simulink model "Running_mex_SIMULINK_PID"  (R2020a)
settings: Solver=VariableStepAuto  StartTime=0.0  StopTime=inf  RelTol=1e-3
values from neighbouring files (symbols this model uses):
  angdes = [0 0 0]    [simulink_run_file.m]
  Kd = .105    (= 0.105)    [simulink_run_file.m]
  Kint = 0.01    [simulink_run_file.m]
  Kint_time = .5    (= 0.5)    [simulink_run_file.m]
  Kp = .065    (= 0.065)    [simulink_run_file.m]
  refresh = .005    (= 0.005)    [simulink_run_file.m]
  Tfinal_master = refresh*NumSteps    [simulink_run_file.m]
  Tmax = 2/1000    (= 0.002)    [simulink_run_file.m]
undefined symbols (not defined in the file or in its folder): get_initial_inputs
settings Model: Creator=hoddid  LastModifiedBy=hoddid

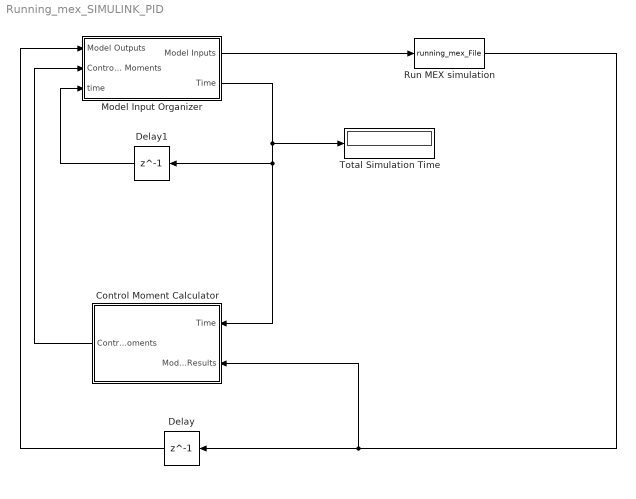
== system Running_mex_SIMULINK_PID ==
  Control Moment Calculator : Subsystem
  Delay : Delay  DelayLength=1
  Delay1 : Delay  DelayLength=1
  Model Input Organizer : Subsystem
  Run MEX simulation : MATLABFcn  MATLABFcn=running_mex_File  OutputDimensions=[1 32]  Output1D=off
  Total Simulation Time : Display
  wires:
  Model Input Organizer/1(Model Inputs) -> Run MEX simulation/1
  Delay/1 -> Model Input Organizer/1(Model Outputs)
  Delay1/1 -> Model Input Organizer/3(time)
  Control Moment Calculator/1(Control Moments) -> Model Input Organizer/2(Control Moments)
  Run MEX simulation/1 -> Control Moment Calculator/2(Model Results), Delay/1
  Model Input Organizer/2(Time) -> Delay1/1, Control Moment Calculator/1(Time), Total Simulation Time/1

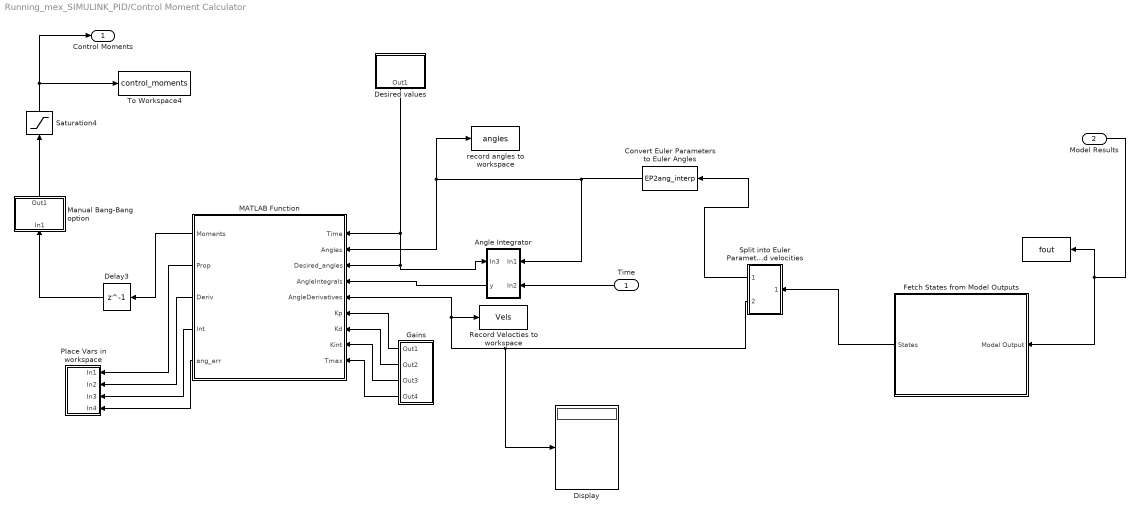
== system Running_mex_SIMULINK_PID/Control Moment Calculator ==
  Time : Inport
  Model Results : Inport  Port=2
  " " : ToWorkspace  VariableName=fout  SampleTime=-1
      settings: Save2DSignal=2-D array (concatenate along first dimension)
  Angle Integrator : Subsystem
      settings: PortSchema="{\"entries\":[{\"content\":{\"sides\":[{\"content\":{\"connectorIds\":[\"In1\",\"In2\"]},\"type\":\"ConnectorPlacement.EquallySpacedRectSide\",\"uuid\":\"d6ec8e57-2ce1-4645-aea4-117e31adf036\"},{\"content\":{\"connectorIds\":[\"In3\",\"Out1\"],\"side\":\"RIGHT\"},\"type\":\"ConnectorPlacement.EquallySpacedRectSide\",\"uuid\":\"9aa7eeac-e178-4ab4-b442-dff06071aa4f\"},{\"content\":{\"connectorIds\":[],\"side\":\"TOP\"},\"type\":\"ConnectorPlacement.EquallySpacedRectSide\",\"uuid\":\"a38c2929-0d18-4e94-afd9-f74ecc2586ec\"}]},\"type\":\"ConnectorPlacement.EquallySpacedConnector\",\"uuid\":\"06fa8231-8b3e-4404-bfb9-ddb3e7039ceb\"}],\"packageUris\":[\"http://schema.mathworks.com/mf0/Connector/19700101\"],\"version\":\"1.0\"}"
  Convert Euler Parameters to Euler Angles : MATLABFcn  MATLABFcn=EP2ang_interp
  Delay3 : Delay  DelayLength=1
  Desired values : Subsystem
  Display : Display
  Fetch States from Model Outputs : Subsystem
  Gains : Subsystem
  MATLAB Function : MATLAB Function  TreatAsAtomicUnit=on
  Manual Bang-Bang option : Subsystem
  Place Vars in workspace : Subsystem
  Record Velocties to workspace : ToWorkspace  VariableName=Vels  SampleTime=-1
      settings: Save2DSignal=2-D array (concatenate along first dimension)
  Saturation4 : Saturate  UpperLimit=Tmax  LowerLimit=-Tmax
  Split into Euler Parameters and velocities : Subsystem
  To Workspace4 : ToWorkspace  VariableName=control_moments  SampleTime=-1
      settings: Save2DSignal=2-D array (concatenate along first dimension)
  record angles to workspace : ToWorkspace  VariableName=angles  SampleTime=-1
      settings: Save2DSignal=2-D array (concatenate along first dimension)
  Control Moments : Outport
  wires:
  Desired values/1(Out1) -> Angle Integrator/3(In3), MATLAB Function/3(Desired_angles), MATLAB Function/1(Time)
  Model Results/1 -> " "/1, Fetch States from Model Outputs/1(Model Output)
  Angle Integrator/1(y) -> MATLAB Function/4(AngleIntegrals)
  MATLAB Function/1(Moments) -> Delay3/1
  MATLAB Function/2(Prop) -> Place Vars in workspace/1(In1)
  MATLAB Function/3(Deriv) -> Place Vars in workspace/2(In2)
  MATLAB Function/4(Int) -> Place Vars in workspace/3(In3)
  MATLAB Function/5(ang_err) -> Place Vars in workspace/4(In4)
  Gains/1(Out1) -> MATLAB Function/6(Kp)
  Gains/2(Out2) -> MATLAB Function/7(Kd)
  Gains/3(Out3) -> MATLAB Function/8(Kint)
  Gains/4(Out4) -> MATLAB Function/9(Tmax)
  Split into Euler Parameters and velocities/2(Out2) -> Display/1, Record Velocties to workspace/1, MATLAB Function/5(AngleDerivatives)
  Fetch States from Model Outputs/1(States) -> Split into Euler Parameters and velocities/1(In1)
  Split into Euler Parameters and velocities/1(Out1) -> Convert Euler Parameters to Euler Angles/1
  Saturation4/1 -> Control Moments/1, To Workspace4/1
  Time/1 -> Angle Integrator/2(In2)
  Convert Euler Parameters to Euler Angles/1 -> record angles to workspace/1, MATLAB Function/2(Angles), Angle Integrator/1(In1)
  Delay3/1 -> Manual Bang-Bang option/1(In1)
  Manual Bang-Bang option/1(Out1) -> Saturation4/1

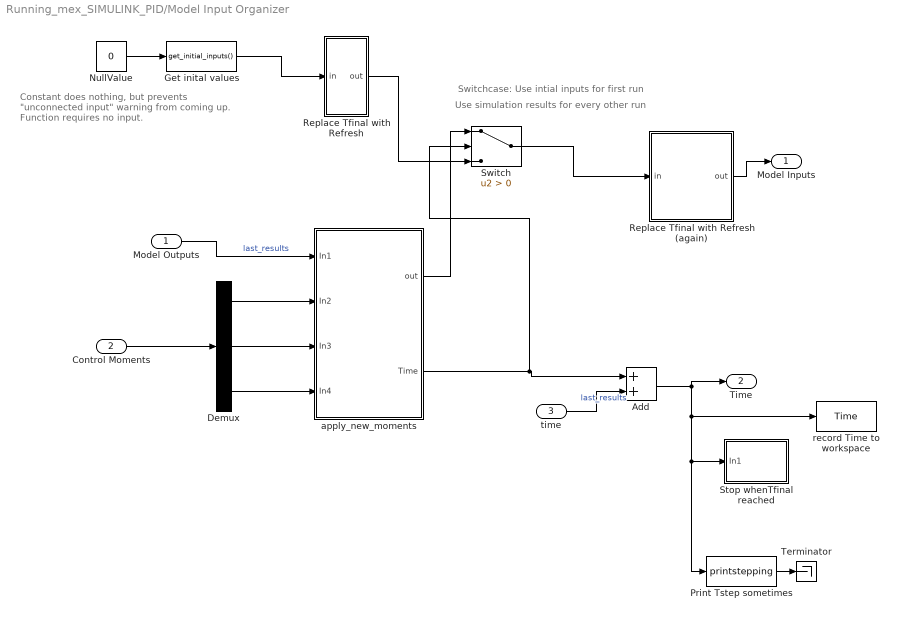
== system Running_mex_SIMULINK_PID/Model Input Organizer ==
  note: Use simulation results for every other run
  note: Switchcase: Use intial inputs for first run
  note: Constant does nothing, but prevents
      | "unconnected input" warning from coming up.
      | Function requires no input.
  Model Outputs : Inport
  Control Moments : Inport  Port=2
  time : Inport  Port=3
  Add : Sum
  Demux : Demux  Outputs=3
  "Get inital values " : MATLABFcn  MATLABFcn=get_initial_inputs()
  NullValue : Constant  Value=0
  Print Tstep sometimes : MATLABFcn  MATLABFcn=printstepping
  Replace Tfinal with Refresh : Subsystem
  Replace Tfinal with Refresh (again) : Subsystem
  Stop whenTfinal reached : Subsystem
      settings: PortSchema="{\"entries\":[{\"content\":{\"sides\":[{\"content\":{\"connectorIds\":[]},\"type\":\"ConnectorPlacement.EquallySpacedRectSide\",\"uuid\":\"b8031d13-d17c-4f9a-b5f8-92da6927a3ba\"},{\"content\":{\"connectorIds\":[],\"side\":\"RIGHT\"},\"type\":\"ConnectorPlacement.EquallySpacedRectSide\",\"uuid\":\"11a71682-1cdb-45f2-b8b8-d175538f4c28\"},{\"content\":{\"connectorIds\":[\"In1\"],\"side\":\"TOP\"},\"type\":\"ConnectorPlacement.EquallySpacedRectSide\",\"uuid\":\"ae57efda-2ecd-443a-aa6f-cfe1c35dec26\"}]},\"type\":\"ConnectorPlacement.EquallySpacedConnector\",\"uuid\":\"64a769af-a08f-48b5-9fd8-ee733c537d04\"}],\"packageUris\":[\"http://schema.mathworks.com/mf0/Connector/19700101\"],\"version\":\"1.0\"}"
  Switch : Switch  Criteria=u2 > Threshold
  Terminator : Terminator
  apply_new_moments : Subsystem
  record Time to workspace : ToWorkspace  VariableName=Time  SampleTime=-1
      settings: Save2DSignal=2-D array (concatenate along first dimension)
  Model Inputs : Outport
  Time : Outport  Port=2
  wires:
  Model Outputs/1 -> apply_new_moments/1(In1)  "last_results"
  apply_new_moments/1(out) -> Switch/1
  apply_new_moments/2(Time) -> Switch/2, Add/1
  time/1 -> Add/2  "last_results"
  Add/1 -> Time/1, Stop whenTfinal reached/1(In1), Print Tstep sometimes/1, record Time to workspace/1
  Switch/1 -> Replace Tfinal with Refresh (again)/1(in)
  "Get inital values "/1 -> Replace Tfinal with Refresh/1(in)
  Replace Tfinal with Refresh/1(out) -> Switch/3
  Replace Tfinal with Refresh (again)/1(out) -> Model Inputs/1
  NullValue/1 -> "Get inital values "/1
  Control Moments/1 -> Demux/1
  Demux/1 -> apply_new_moments/2(In2)
  Demux/2 -> apply_new_moments/3(In3)
  Demux/3 -> apply_new_moments/4(In4)
  Print Tstep sometimes/1 -> Terminator/1

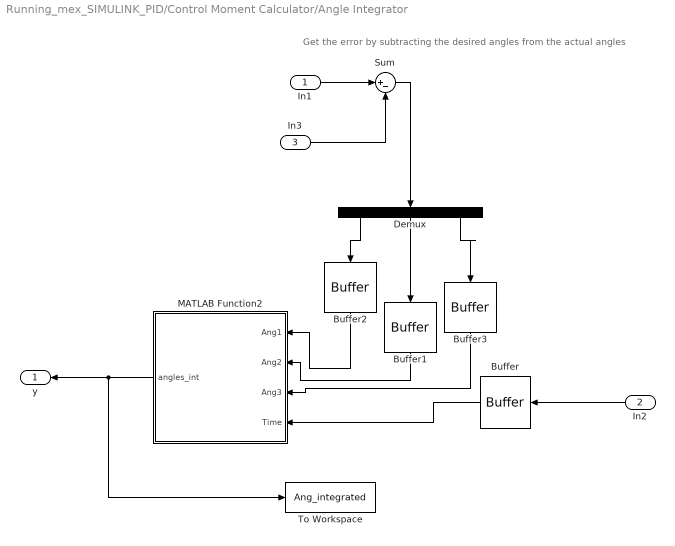
== system Running_mex_SIMULINK_PID/Control Moment Calculator/Angle Integrator ==
  note: Get the error by subtracting the desired angles from the actual angles
  In1 : Inport
  In2 : Inport  Port=2  SampleTime=refresh
  In3 : Inport  Port=3  SampleTime=refresh
  Buffer{,1..3} (4 alike) : Buffer  N=round(Kint_time*(1/refresh))  V=round(Kint_time*(1/refresh))-1  OutputFrames=off
  Demux : Demux  Outputs=3
  MATLAB Function2 : MATLAB Function  TreatAsAtomicUnit=on
  Sum : Sum  Inputs=|+-
  To Workspace : ToWorkspace  VariableName=Ang_integrated  SampleTime=-1
      settings: Save2DSignal=2-D array (concatenate along first dimension)
  y : Outport
  wires:
  Buffer/1 -> MATLAB Function2/4(Time)
  MATLAB Function2/1(angles_int) -> To Workspace/1, y/1
  Demux/2 -> Buffer1/1
  Demux/1 -> Buffer2/1
  Demux/3 -> Buffer3/1
  Buffer2/1 -> MATLAB Function2/1(Ang1)
  Buffer1/1 -> MATLAB Function2/2(Ang2)
  Buffer3/1 -> MATLAB Function2/3(Ang3)
  In2/1 -> Buffer/1
  In1/1 -> Sum/1
  In3/1 -> Sum/2
  Sum/1 -> Demux/1

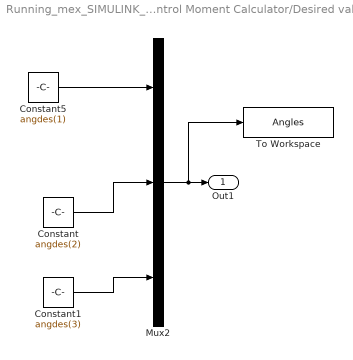
== system Running_mex_SIMULINK_PID/Control Moment Calculator/Desired values ==
  Constant : Constant  Value=angdes(2)
  Constant1 : Constant  Value=angdes(3)
  Constant5 : Constant  Value=angdes(1)
  Mux2 : Mux  Inputs=3
  To Workspace : ToWorkspace  VariableName=Angles  SaveFormat=Timeseries  SampleTime=-1
  Out1 : Outport
  wires:
  Constant1/1 -> Mux2/3
  Constant5/1 -> Mux2/1
  Mux2/1 -> To Workspace/1, Out1/1
  Constant/1 -> Mux2/2

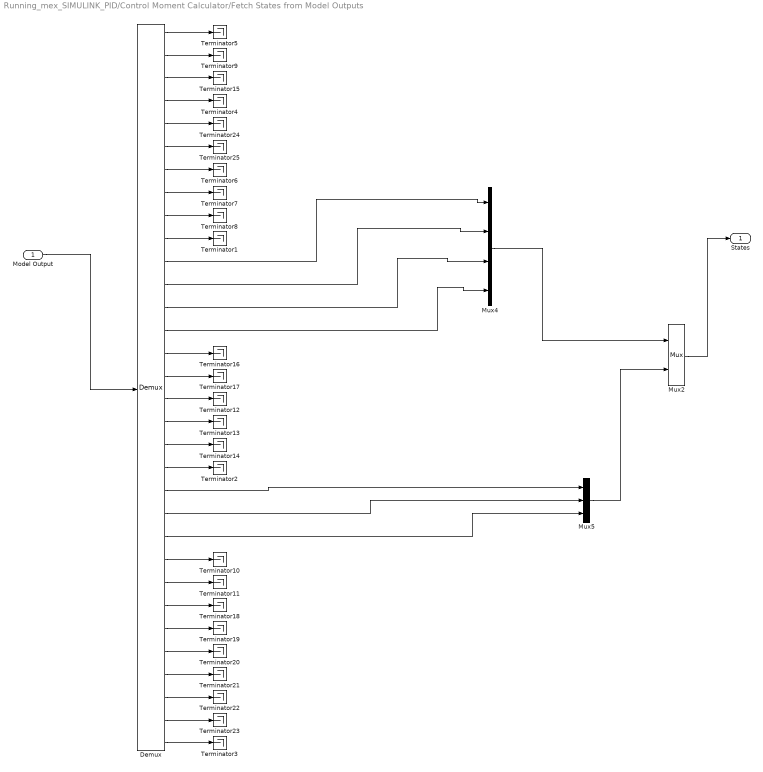
== system Running_mex_SIMULINK_PID/Control Moment Calculator/Fetch States from Model Outputs ==
  Model Output : Inport
  Demux : Demux  Outputs=32
  Mux2 : Mux  Inputs=2
  Mux4 : Mux
  Mux5 : Mux  Inputs=3
  Terminator{1..25} (25 alike) : Terminator
  States : Outport
  wires:
  Demux/15 -> Terminator16/1
  Demux/26 -> Terminator18/1
  Demux/30 -> Terminator22/1
  Demux/14 -> Mux4/4
  Demux/25 -> Terminator11/1
  Demux/29 -> Terminator21/1
  Mux2/1 -> States/1
  Demux/28 -> Terminator20/1
  Demux/24 -> Terminator10/1
  Demux/17 -> Terminator12/1
  Demux/18 -> Terminator13/1
  Demux/7 -> Terminator6/1
  Demux/9 -> Terminator8/1
  Demux/31 -> Terminator23/1
  Demux/27 -> Terminator19/1
  Demux/19 -> Terminator14/1
  Model Output/1 -> Demux/1
  Mux5/1 -> Mux2/2
  Demux/8 -> Terminator7/1
  Demux/23 -> Mux5/3
  Mux4/1 -> Mux2/1
  Demux/16 -> Terminator17/1
  Demux/13 -> Mux4/3
  Demux/12 -> Mux4/2
  Demux/11 -> Mux4/1
  Demux/10 -> Terminator1/1
  Demux/22 -> Mux5/2
  Demux/21 -> Mux5/1
  Demux/20 -> Terminator2/1
  Demux/32 -> Terminator3/1
  Demux/1 -> Terminator5/1
  Demux/2 -> Terminator9/1
  Demux/3 -> Terminator15/1
  Demux/4 -> Terminator4/1
  Demux/6 -> Terminator25/1
  Demux/5 -> Terminator24/1

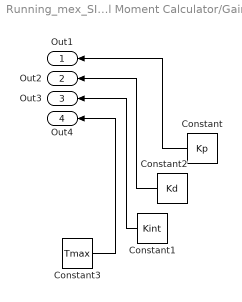
== system Running_mex_SIMULINK_PID/Control Moment Calculator/Gains ==
  Constant : Constant  Value=Kp
  Constant1 : Constant  Value=Kint
  Constant2 : Constant  Value=Kd
  Constant3 : Constant  Value=Tmax
  Out1 : Outport
  Out2 : Outport  Port=2
  Out3 : Outport  Port=3
  Out4 : Outport  Port=4
  wires:
  Constant2/1 -> Out2/1
  Constant3/1 -> Out4/1
  Constant/1 -> Out1/1
  Constant1/1 -> Out3/1

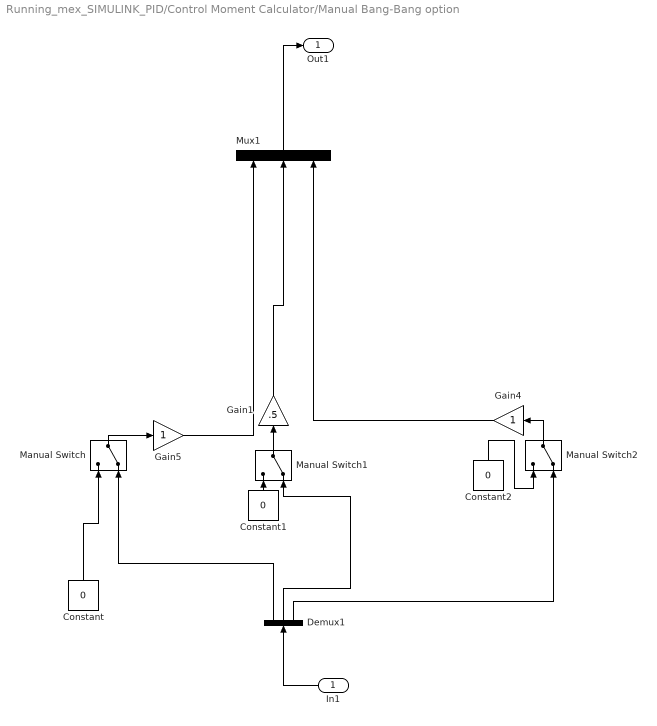
== system Running_mex_SIMULINK_PID/Control Moment Calculator/Manual Bang-Bang option ==
  In1 : Inport
  Constant : Constant  Value=0
  Constant1 : Constant  Value=0
  Constant2 : Constant  Value=0
  Demux1 : Demux  Outputs=3
  Gain1 : Gain  Gain=.5
  Gain4 : Gain
  Gain5 : Gain
  Manual Switch : ManualSwitch  CurrentSetting=0
  Manual Switch1 : ManualSwitch  CurrentSetting=0
  Manual Switch2 : ManualSwitch  CurrentSetting=0
  Mux1 : Mux  Inputs=3
  Out1 : Outport
  wires:
  Demux1/1 -> Manual Switch/2
  Mux1/1 -> Out1/1
  Constant2/1 -> Manual Switch2/1
  Manual Switch2/1 -> Gain4/1
  Demux1/3 -> Manual Switch2/2
  Demux1/2 -> Manual Switch1/2
  Constant1/1 -> Manual Switch1/1
  In1/1 -> Demux1/1
  Manual Switch/1 -> Gain5/1
  Gain4/1 -> Mux1/3
  Manual Switch1/1 -> Gain1/1
  Constant/1 -> Manual Switch/1
  Gain5/1 -> Mux1/1
  Gain1/1 -> Mux1/2

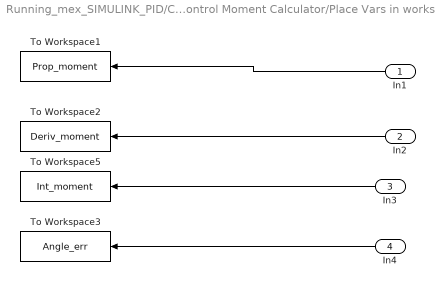
== system Running_mex_SIMULINK_PID/Control Moment Calculator/Place Vars in workspace ==
  In1 : Inport
  In2 : Inport  Port=2
  In3 : Inport  Port=3
  In4 : Inport  Port=4
  To Workspace1 : ToWorkspace  VariableName=Prop_moment  SampleTime=-1
      settings: Save2DSignal=2-D array (concatenate along first dimension)
  To Workspace2 : ToWorkspace  VariableName=Deriv_moment  SampleTime=-1
      settings: Save2DSignal=2-D array (concatenate along first dimension)
  To Workspace3 : ToWorkspace  VariableName=Angle_err  SampleTime=-1
      settings: Save2DSignal=2-D array (concatenate along first dimension)
  To Workspace5 : ToWorkspace  VariableName=Int_moment  SampleTime=-1
      settings: Save2DSignal=2-D array (concatenate along first dimension)
  wires:
  In3/1 -> To Workspace5/1
  In1/1 -> To Workspace1/1
  In2/1 -> To Workspace2/1
  In4/1 -> To Workspace3/1

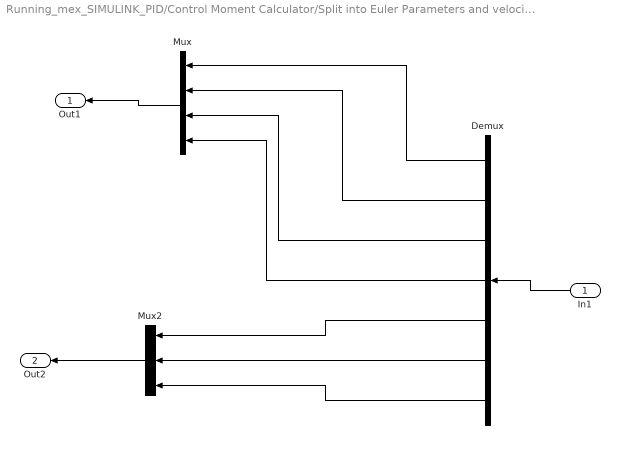
== system Running_mex_SIMULINK_PID/Control Moment Calculator/Split into Euler Parameters and velocities ==
  In1 : Inport
  Demux : Demux  Outputs=7
  Mux : Mux
  Mux2 : Mux  Inputs=3
  Out1 : Outport
  Out2 : Outport  Port=2
  wires:
  Demux/5 -> Mux2/1
  Demux/4 -> Mux/4
  In1/1 -> Demux/1
  Demux/2 -> Mux/2
  Demux/3 -> Mux/3
  Demux/6 -> Mux2/2
  Demux/7 -> Mux2/3
  Mux2/1 -> Out2/1
  Demux/1 -> Mux/1
  Mux/1 -> Out1/1

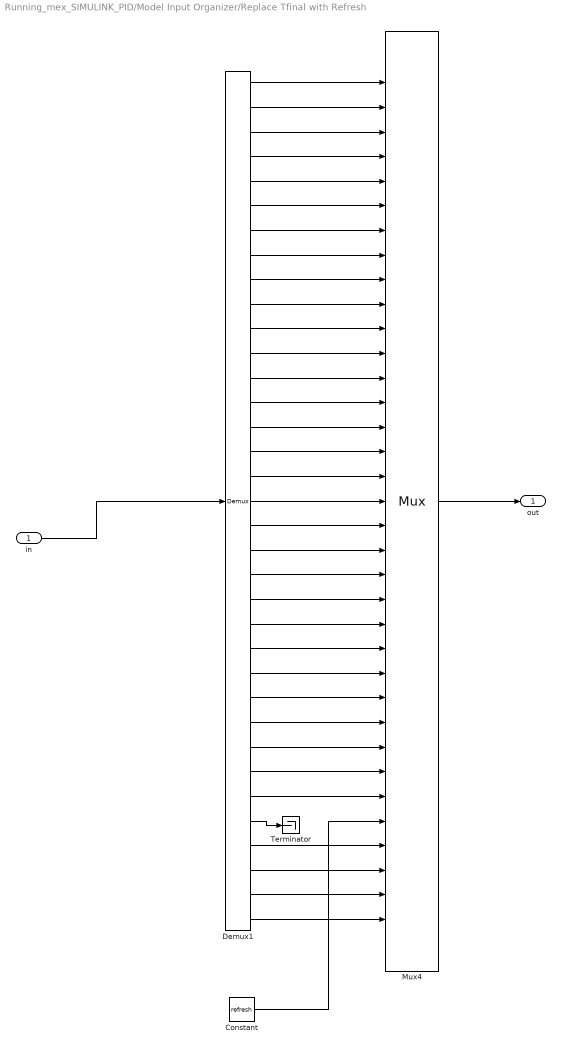
== system Running_mex_SIMULINK_PID/Model Input Organizer/Replace Tfinal with Refresh ==
  in : Inport
  Constant : Constant  Value=refresh
  Demux1 : Demux  Outputs=35
  Mux4 : Mux  Inputs=35
  Terminator : Terminator
  out : Outport  OutDataTypeStr=double
  wires:
  in/1 -> Demux1/1
  Mux4/1 -> out/1
  Demux1/1 -> Mux4/1
  Demux1/2 -> Mux4/2
  Demux1/3 -> Mux4/3
  Demux1/4 -> Mux4/4
  Demux1/5 -> Mux4/5
  Demux1/6 -> Mux4/6
  Demux1/7 -> Mux4/7
  Demux1/8 -> Mux4/8
  Demux1/9 -> Mux4/9
  Demux1/10 -> Mux4/10
  Demux1/11 -> Mux4/11
  Demux1/12 -> Mux4/12
  Demux1/13 -> Mux4/13
  Demux1/14 -> Mux4/14
  Demux1/15 -> Mux4/15
  Demux1/16 -> Mux4/16
  Demux1/17 -> Mux4/17
  Demux1/18 -> Mux4/18
  Demux1/19 -> Mux4/19
  Demux1/20 -> Mux4/20
  Demux1/21 -> Mux4/21
  Demux1/22 -> Mux4/22
  Demux1/23 -> Mux4/23
  Demux1/24 -> Mux4/24
  Demux1/25 -> Mux4/25
  Demux1/26 -> Mux4/26
  Demux1/27 -> Mux4/27
  Demux1/28 -> Mux4/28
  Demux1/29 -> Mux4/29
  Constant/1 -> Mux4/31
  Demux1/31 -> Terminator/1
  Demux1/35 -> Mux4/35
  Demux1/34 -> Mux4/34
  Demux1/33 -> Mux4/33
  Demux1/32 -> Mux4/32
  Demux1/30 -> Mux4/30

== system Running_mex_SIMULINK_PID/Model Input Organizer/Replace Tfinal with Refresh (again) ==
  in : Inport
  Constant : Constant  Value=refresh
  Demux1 : Demux  Outputs=35
  Mux4 : Mux  Inputs=35
  Terminator : Terminator
  out : Outport  OutDataTypeStr=double
  wires:
  in/1 -> Demux1/1
  Mux4/1 -> out/1
  Demux1/1 -> Mux4/1
  Demux1/2 -> Mux4/2
  Demux1/3 -> Mux4/3
  Demux1/4 -> Mux4/4
  Demux1/5 -> Mux4/5
  Demux1/6 -> Mux4/6
  Demux1/7 -> Mux4/7
  Demux1/8 -> Mux4/8
  Demux1/9 -> Mux4/9
  Demux1/10 -> Mux4/10
  Demux1/11 -> Mux4/11
  Demux1/12 -> Mux4/12
  Demux1/13 -> Mux4/13
  Demux1/14 -> Mux4/14
  Demux1/15 -> Mux4/15
  Demux1/16 -> Mux4/16
  Demux1/17 -> Mux4/17
  Demux1/18 -> Mux4/18
  Demux1/19 -> Mux4/19
  Demux1/20 -> Mux4/20
  Demux1/21 -> Mux4/21
  Demux1/22 -> Mux4/22
  Demux1/23 -> Mux4/23
  Demux1/24 -> Mux4/24
  Demux1/25 -> Mux4/25
  Demux1/26 -> Mux4/26
  Demux1/27 -> Mux4/27
  Demux1/28 -> Mux4/28
  Demux1/29 -> Mux4/29
  Constant/1 -> Mux4/31
  Demux1/31 -> Terminator/1
  Demux1/35 -> Mux4/35
  Demux1/34 -> Mux4/34
  Demux1/33 -> Mux4/33
  Demux1/32 -> Mux4/32
  Demux1/30 -> Mux4/30

== system Running_mex_SIMULINK_PID/Model Input Organizer/Stop whenTfinal reached ==
  note: Stop the simulation
  note: If the simulation time is greater than or equal to the final simulation time
  In1 : Inport
  Constant4 : Constant  Value=0
  Constant5 : Constant
  Stop Simulation : Stop
  Switch1 : Switch  Criteria=u2 > Threshold  Threshold=Tfinal_master-(refresh/2)
  wires:
  Constant4/1 -> Switch1/3
  In1/1 -> Switch1/2
  Switch1/1 -> Stop Simulation/1
  Constant5/1 -> Switch1/1

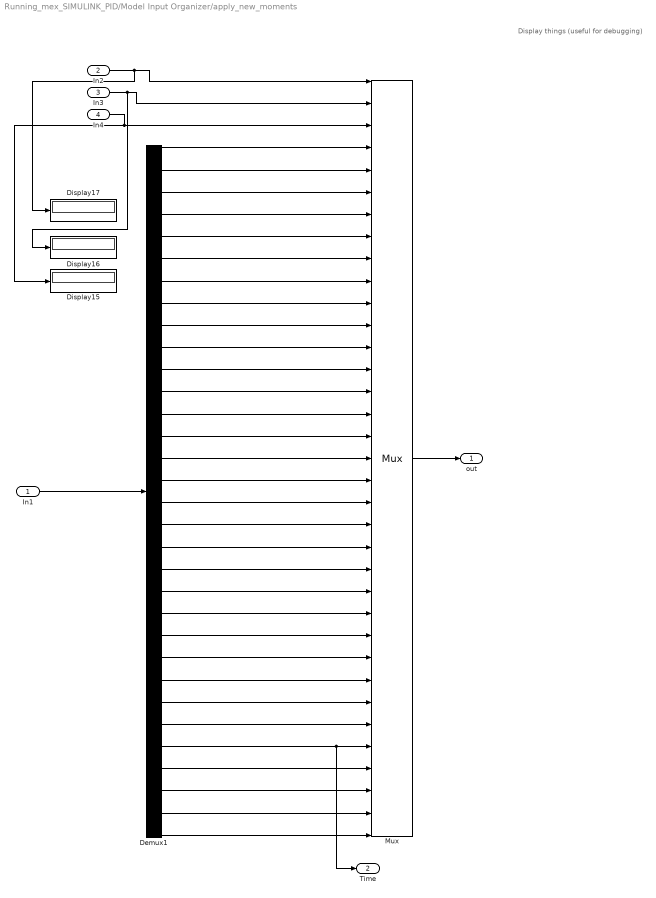
== system Running_mex_SIMULINK_PID/Model Input Organizer/apply_new_moments ==
  note: Display things (useful for debugging)
  In1 : Inport
  In2 : Inport  Port=2
  In3 : Inport  Port=3
  In4 : Inport  Port=4
  Demux1 : Demux  Outputs=32
  Display15 : Display
  Display16 : Display
  Display17 : Display
  Mux : Mux  Inputs=35
  out : Outport  OutDataTypeStr=double
  Time : Outport  Port=2
  wires:
  In1/1 -> Demux1/1
  In4/1 -> Mux/3, Display15/1
  In3/1 -> Display16/1, Mux/2
  In2/1 -> Display17/1, Mux/1
  Mux/1 -> out/1
  Demux1/2 -> Mux/5
  Demux1/3 -> Mux/6
  Demux1/4 -> Mux/7
  Demux1/5 -> Mux/8
  Demux1/6 -> Mux/9
  Demux1/7 -> Mux/10
  Demux1/8 -> Mux/11
  Demux1/9 -> Mux/12
  Demux1/10 -> Mux/13
  Demux1/11 -> Mux/14
  Demux1/12 -> Mux/15
  Demux1/13 -> Mux/16
  Demux1/14 -> Mux/17
  Demux1/15 -> Mux/18
  Demux1/16 -> Mux/19
  Demux1/17 -> Mux/20
  Demux1/18 -> Mux/21
  Demux1/19 -> Mux/22
  Demux1/20 -> Mux/23
  Demux1/21 -> Mux/24
  Demux1/22 -> Mux/25
  Demux1/23 -> Mux/26
  Demux1/24 -> Mux/27
  Demux1/25 -> Mux/28
  Demux1/26 -> Mux/29
  Demux1/27 -> Mux/30
  Demux1/28 -> Time/1, Mux/31
  Demux1/29 -> Mux/32
  Demux1/30 -> Mux/33
  Demux1/31 -> Mux/34
  Demux1/32 -> Mux/35
  Demux1/1 -> Mux/4

== matlab function Running_mex_SIMULINK_PID/Control Moment Calculator/MATLAB Function ==
  data: Time input; Angles input; Desired_angles input; Moments output; AngleIntegrals input; AngleDerivatives input; Kp input; Kd input; Kint input; Prop output; Deriv output; Int output; ang_err output; Tmax input
function [Moments,Prop,Deriv,Int,ang_err] = PIDcontroller(Time,Angles,Desired_angles,AngleIntegrals,AngleDerivatives,Kp,Kd,Kint,Tmax)
% This function creates control moments via PID control
ang_err = Angles-Desired_angles;



%% Create moments 
%this if statment is neccisary as there is no integral term at time = zero
if Time == 0
    Prop = [-Kp*ang_err(1),Kp*ang_err(2),Kp*ang_err(3)];
    Deriv = [Kd*(AngleDerivatives(1)),Kd*(AngleDerivatives(2)),-Kd*(AngleDerivatives(3))];
    Int = [0,0,0];
else 
    Prop = [-Kp*ang_err(1),Kp*ang_err(2),Kp*ang_err(3)];
    Deriv = [Kd*(AngleDerivatives(1)),Kd*(AngleDerivatives(2)),-Kd*(AngleDerivatives(3))];
    Int = [-Kint*(AngleIntegrals(1)),Kint*(AngleIntegrals(2)),Kint*(AngleIntegrals(3))];
end

%Sum different components of the moment
U1 = Prop(1) + Deriv(1) + Int(1);
U2 = Prop(2) + Deriv(2) + Int(2);
U3 = Prop(3) + Deriv(3) + Int(3);

Moments = [U1,U2,-U3]; %note the -U3, as the model defines the third axis 'Upside down' compared to the other 2
end

== matlab function Running_mex_SIMULINK_PID/Control Moment Calculator/Angle Integrator/MATLAB Function2 ==
  data: Ang1 input; angles_int output; Ang2 input; Ang3 input; Time input
function angles_int = Angle_integrator(Ang1,Ang2,Ang3,Time)
% This function creates the integral of the angular errors via trapz
Time_tointegrate = Time;
%Integrate Via trapz
int1 = trapz(Time_tointegrate,Ang1);
int2 = trapz(Time_tointegrate,Ang2);
int3 = trapz(Time_tointegrate,Ang3);

%return integral of errors
angles_int = [int1,int2,int3];

end
